simulink model "three_level_SPWM_3ph_VSI"  (R2022b)
settings: Solver=FixedStepAuto  StartTime=0.0  StopTime=0.2  RelTol=1e-3
libraries: spsIGBTDiodeLib x18, spsDiodeLib x6, spsSeriesRLCBranchLib x6, spsDCVoltageSourceLib x4, spsVoltageMeasurementLib x4, spsGroundLib x2, simulink x2, spsTriangleGeneratorLib x1, spspowerguiLib x1
settings Model: Creator=jack  LastModifiedBy=jackyeh
settings DataIOCC: InspectSignalLogs=on

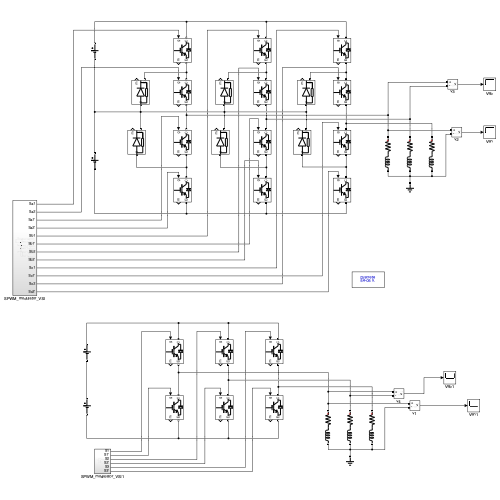
[thumbnail: Simulink's stored preview of the top-level diagram]
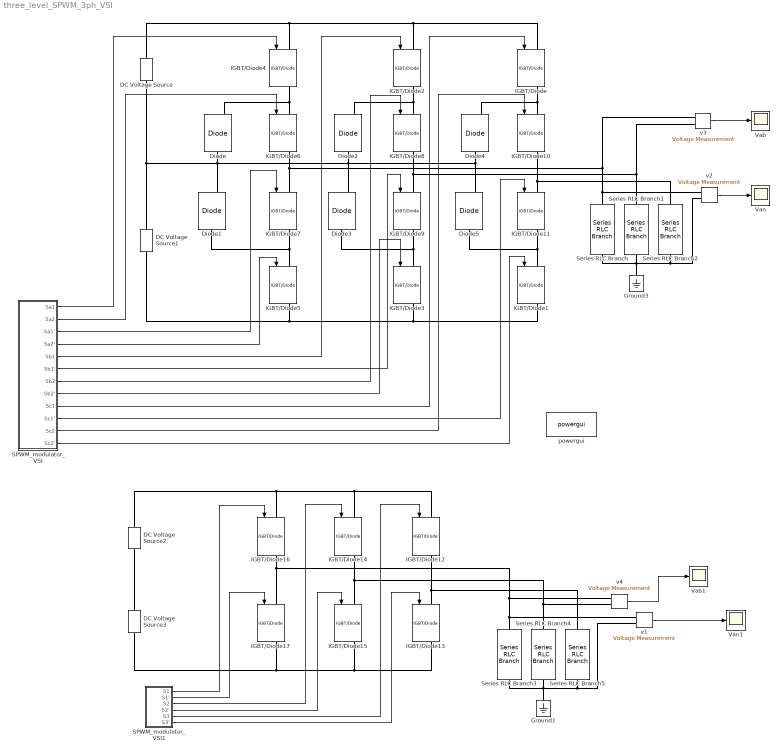
== system three_level_SPWM_3ph_VSI ==
  DC Voltage Source{,1..3} (4 alike) : spsDCVoltageSourceLib/DC Voltage Source  Amplitude=100  Measurements=None
  Diode{,1..5} (6 alike) : spsDiodeLib/Diode  Ron=0.001  Lon=0  Vf=0.8  IC=0  UseSnubber=0  Rs=500  Cs=250e-9  Measurements=on
  Ground1 : spsGroundLib/Ground  LConnTagsString=a
  Ground3 : spsGroundLib/Ground  LConnTagsString=a
  IGBT/Diode{,1..17} (18 alike) : spsIGBTDiodeLib/IGBT//Diode  Ron=1e-3  Rs=1e5  Cs=inf  Measurements=on
  SPWM_modulator_VSI : Subsystem
  SPWM_modulator_VSI1 : Subsystem
  Series RLC Branch{,1..5} (6 alike) : spsSeriesRLCBranchLib/Series RLC Branch  LConnTagsString=__new0  RConnTagsString=__new0  BranchType=RL  Resistance=5  Inductance=150e-3  SetiL0=off  InitialCurrent=0  Capacitance=0  Setx0=off  InitialVoltage=0  Measurements=None
  Vab : Scope
  Vab1 : Scope
  Van : Scope
  Van1 : Scope
  powergui : spspowerguiLib/powergui  Priority=1  SimulationMode=Discrete  SampleTime=50e-6  frequency=60  Iterations=50  frequencyindice=0  Pbase=100e6  ErrMax=1e-4  UnitsV=kV  UnitsW=MW  buscounter=0  FunctionMessages=off  echomessages=off  EnableUseOfTLC=off  CurrentSourceSwitches=off  DisableSnubberDevices=off  DisableRonSwitches=off  DisableVfSwitches=off  DisplayEquations=off  AutomaticDiscreteSolvers=off  SolverType=Tustin/Backward Euler (TBE)  Interpol=off  ExternalGateDelay=off  methode=off  Ts=100  x0status=blocks  SPID=on  SwTol=0  HookPort=off  NonlinearTolerance=1e-4  nMaxIteration=100  ContinueOnMaxIteration=off  RestoreLinks=warning  ResistiveCurrentMeasurement=off  Frange=[0:2:500]  Ylog=off  Xlog=on  ShowGrid=off  save=off  variable=ZData  structure=0  ZoomFFT=off  StartTime=0.0  cycles=1  DisplayStyle=1  fundamental=60  FreqAxis=off  MaxFrequency=1000  frequencyindicesteady=1  RmsSteady=1  display=off
  v{1..4} (4 alike) : spsVoltageMeasurementLib/Voltage Measurement  PhasorSimulation=off  OutputType=Complex  PSBequivalent=0
  wires:
  v2/1 -> Van/1
  v3/1 -> Vab/1
  SPWM_modulator_VSI/1(Sa1) -> IGBT/Diode4/1
  SPWM_modulator_VSI/2(Sa2) -> IGBT/Diode6/1
  SPWM_modulator_VSI/3(Sa1') -> IGBT/Diode7/1
  SPWM_modulator_VSI/4(Sa2') -> IGBT/Diode5/1
  SPWM_modulator_VSI/5(Sb1) -> IGBT/Diode2/1
  SPWM_modulator_VSI/8(Sb2') -> IGBT/Diode3/1
  SPWM_modulator_VSI/9(Sc1) -> IGBT/Diode/1
  SPWM_modulator_VSI/10(Sc1') -> IGBT/Diode11/1
  SPWM_modulator_VSI/11(Sc2) -> IGBT/Diode10/1
  SPWM_modulator_VSI/12(Sc2') -> IGBT/Diode1/1
  SPWM_modulator_VSI/6(Sb1') -> IGBT/Diode9/1
  SPWM_modulator_VSI/7(Sb2) -> IGBT/Diode8/1
  SPWM_modulator_VSI1/6(S3') -> IGBT/Diode13/1
  v4/1 -> Vab1/1
  SPWM_modulator_VSI1/3(S2) -> IGBT/Diode14/1
  SPWM_modulator_VSI1/4(S2') -> IGBT/Diode15/1
  SPWM_modulator_VSI1/1(S1) -> IGBT/Diode16/1
  v1/1 -> Van1/1
  SPWM_modulator_VSI1/2(S1') -> IGBT/Diode17/1
  SPWM_modulator_VSI1/5(S3) -> IGBT/Diode12/1
  connections:
  DC Voltage Source1/LConn1 -- IGBT/Diode1/RConn1 -- IGBT/Diode3/RConn1 -- IGBT/Diode5/RConn1
  DC Voltage Source/RConn1 -- IGBT/Diode4/LConn1 -- IGBT/Diode2/LConn1 -- IGBT/Diode/LConn1
  IGBT/Diode7/LConn1 -- v3/LConn1 -- Series RLC Branch/LConn1 -- v2/LConn1 -- IGBT/Diode6/RConn1
  DC Voltage Source1/RConn1 -- Diode5/RConn1 -- Diode4/LConn1 -- Diode3/RConn1 -- Diode2/LConn1 -- Diode1/RConn1 -- Diode/LConn1 -- DC Voltage Source/LConn1
  Series RLC Branch1/RConn1 -- v2/LConn2 -- Series RLC Branch2/RConn1 -- Series RLC Branch/RConn1 -- Ground3/LConn1
  IGBT/Diode7/RConn1 -- Diode1/LConn1 -- IGBT/Diode5/LConn1
  IGBT/Diode6/LConn1 -- Diode/RConn1 -- IGBT/Diode4/RConn1
  IGBT/Diode8/LConn1 -- Diode2/RConn1 -- IGBT/Diode2/RConn1
  IGBT/Diode9/LConn1 -- v3/LConn2 -- Series RLC Branch1/LConn1 -- IGBT/Diode8/RConn1
  IGBT/Diode9/RConn1 -- Diode3/LConn1 -- IGBT/Diode3/LConn1
  IGBT/Diode/RConn1 -- Diode4/RConn1 -- IGBT/Diode10/LConn1
  IGBT/Diode10/RConn1 -- Series RLC Branch2/LConn1 -- IGBT/Diode11/LConn1
  IGBT/Diode11/RConn1 -- Diode5/LConn1 -- IGBT/Diode1/LConn1
  Ground1/LConn1 -- Series RLC Branch4/RConn1 -- v1/LConn2 -- Series RLC Branch5/RConn1 -- Series RLC Branch3/RConn1
  IGBT/Diode12/LConn1 -- DC Voltage Source2/RConn1 -- IGBT/Diode16/LConn1 -- IGBT/Diode14/LConn1
  Series RLC Branch5/LConn1 -- IGBT/Diode13/LConn1 -- IGBT/Diode12/RConn1
  IGBT/Diode15/LConn1 -- IGBT/Diode14/RConn1 -- Series RLC Branch4/LConn1 -- v4/LConn2
  IGBT/Diode15/RConn1 -- IGBT/Diode13/RConn1 -- DC Voltage Source3/LConn1 -- IGBT/Diode17/RConn1
  Series RLC Branch3/LConn1 -- IGBT/Diode16/RConn1 -- IGBT/Diode17/LConn1 -- v4/LConn1 -- v1/LConn1
  DC Voltage Source3/RConn1 -- DC Voltage Source2/LConn1

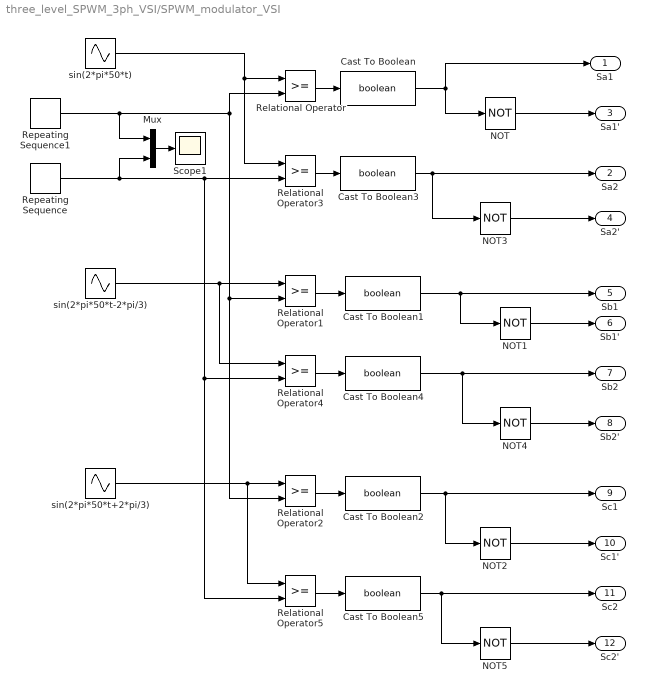
== system three_level_SPWM_3ph_VSI/SPWM_modulator_VSI ==
  Cast To Boolean{,1..5} (6 alike) : DataTypeConversion  OutDataTypeStr=boolean  SaturateOnIntegerOverflow=off  RndMeth=Floor
  Mux : Mux  Inputs=2
  NOT{,1..5} (6 alike) : Logic  Operator=NOT  IconShape=distinctive  AllPortsSameDT=off  OutDataTypeStr=boolean
  Relational Operator{,1..5} (6 alike) : RelationalOperator  OutDataTypeStr=boolean  RndMeth=Simplest  InputSameDT=off
  Repeating Sequence : simulink/Sources/Repeating Sequence  rep_seq_t=[0 0.5 1]/2000  rep_seq_y=[-1 0 -1]
  Repeating Sequence1 : simulink/Sources/Repeating Sequence  rep_seq_t=[0 0.5 1]/2000  rep_seq_y=[0 1 0]
  Scope1 : Scope
  sin(2*pi*50*t) : Sin  Frequency=2*pi*50  SampleTime=0
  sin(2*pi*50*t+2*pi/3) : Sin  Frequency=2*pi*50  Phase=2*pi/3  SampleTime=0
  sin(2*pi*50*t-2*pi/3) : Sin  Frequency=2*pi*50  Phase=-2*pi/3  SampleTime=0
  Sa1 : Outport
  Sa2 : Outport  Port=2
  Sa1' : Outport  Port=3
  Sa2' : Outport  Port=4
  Sb1 : Outport  Port=5
  Sb1' : Outport  Port=6
  Sb2 : Outport  Port=7
  Sb2' : Outport  Port=8
  Sc1 : Outport  Port=9
  Sc1' : Outport  Port=10
  Sc2 : Outport  Port=11
  Sc2' : Outport  Port=12
  wires:
  Relational Operator/1 -> Cast To Boolean/1
  Cast To Boolean/1 -> Sa1/1, NOT/1
  sin(2*pi*50*t)/1 -> Relational Operator3/1, Relational Operator/1
  Relational Operator1/1 -> Cast To Boolean1/1
  Cast To Boolean1/1 -> Sb1/1, NOT1/1
  sin(2*pi*50*t-2*pi/3)/1 -> Relational Operator4/1, Relational Operator1/1
  Relational Operator2/1 -> Cast To Boolean2/1
  sin(2*pi*50*t+2*pi/3)/1 -> Relational Operator5/1, Relational Operator2/1
  Cast To Boolean2/1 -> Sc1/1, NOT2/1
  Relational Operator3/1 -> Cast To Boolean3/1
  Repeating Sequence/1 -> Mux/2, Relational Operator5/2, Relational Operator4/2, Relational Operator3/2
  Cast To Boolean3/1 -> NOT3/1, Sa2/1
  NOT3/1 -> Sa2'/1
  NOT/1 -> Sa1'/1
  Repeating Sequence1/1 -> Mux/1, Relational Operator/2, Relational Operator2/2, Relational Operator1/2
  Relational Operator4/1 -> Cast To Boolean4/1
  NOT1/1 -> Sb1'/1
  Cast To Boolean4/1 -> NOT4/1, Sb2/1
  NOT4/1 -> Sb2'/1
  Relational Operator5/1 -> Cast To Boolean5/1
  NOT2/1 -> Sc1'/1
  Cast To Boolean5/1 -> NOT5/1, Sc2/1
  NOT5/1 -> Sc2'/1
  Mux/1 -> Scope1/1

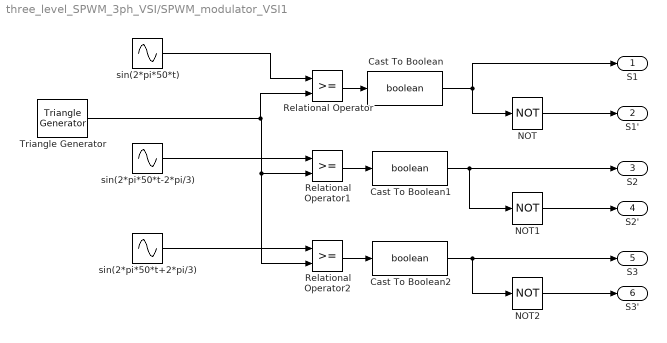
== system three_level_SPWM_3ph_VSI/SPWM_modulator_VSI1 ==
  Cast To Boolean : DataTypeConversion  OutDataTypeStr=boolean  SaturateOnIntegerOverflow=off  RndMeth=Floor
  Cast To Boolean1 : DataTypeConversion  OutDataTypeStr=boolean  SaturateOnIntegerOverflow=off  RndMeth=Floor
  Cast To Boolean2 : DataTypeConversion  OutDataTypeStr=boolean  SaturateOnIntegerOverflow=off  RndMeth=Floor
  NOT : Logic  Operator=NOT  IconShape=distinctive  AllPortsSameDT=off  OutDataTypeStr=boolean
  NOT1 : Logic  Operator=NOT  IconShape=distinctive  AllPortsSameDT=off  OutDataTypeStr=boolean
  NOT2 : Logic  Operator=NOT  IconShape=distinctive  AllPortsSameDT=off  OutDataTypeStr=boolean
  Relational Operator : RelationalOperator  OutDataTypeStr=boolean  RndMeth=Simplest  InputSameDT=off
  Relational Operator1 : RelationalOperator  OutDataTypeStr=boolean  RndMeth=Simplest  InputSameDT=off
  Relational Operator2 : RelationalOperator  OutDataTypeStr=boolean  RndMeth=Simplest  InputSameDT=off
  Triangle Generator : spsTriangleGeneratorLib/Triangle Generator  Freq=2e3  Phase=90  Ts=0
  sin(2*pi*50*t) : Sin  Frequency=2*pi*50  SampleTime=0
  sin(2*pi*50*t+2*pi/3) : Sin  Frequency=2*pi*50  Phase=2*pi/3  SampleTime=0
  sin(2*pi*50*t-2*pi/3) : Sin  Frequency=2*pi*50  Phase=-2*pi/3  SampleTime=0
  S1 : Outport
  S1' : Outport  Port=2
  S2 : Outport  Port=3
  S2' : Outport  Port=4
  S3 : Outport  Port=5
  S3' : Outport  Port=6
  wires:
  NOT/1 -> S1'/1
  Relational Operator/1 -> Cast To Boolean/1
  Cast To Boolean/1 -> S1/1, NOT/1
  Triangle Generator/1 -> Relational Operator/2, Relational Operator2/2, Relational Operator1/2
  sin(2*pi*50*t)/1 -> Relational Operator/1
  Relational Operator1/1 -> Cast To Boolean1/1
  Cast To Boolean1/1 -> S2/1, NOT1/1
  NOT1/1 -> S2'/1
  sin(2*pi*50*t-2*pi/3)/1 -> Relational Operator1/1
  Relational Operator2/1 -> Cast To Boolean2/1
  sin(2*pi*50*t+2*pi/3)/1 -> Relational Operator2/1
  NOT2/1 -> S3'/1
  Cast To Boolean2/1 -> NOT2/1, S3/1
